simulink model "IM_close-loop"  (R2019a)
settings: Solver=FixedStepAuto  StartTime=0.0  StopTime=1  FixedStep=0.00001  RelTol=1e-3
values from neighbouring files (symbols this model uses):
  A1 = [a1 0 a2 0; 0 a1 0 a2; a4 0 a5 0 ; 0 a4 0 a5]    [parametre_IM.m]
  A2 = [0 0 0 a3; 0 0 -a3 0 ; 0 0 0 -1 ; 0 0 1 0]    [parametre_IM.m]
  B = [1/(Ls*sigma) 0; 0 1/(Ls*sigma); 0 0; 0 0]    [parametre_IM.m]
  ClarkConcordia = sqrt(3/2)*[1 -1/2 -1/2; 0 sqrt(3)/2 -sqrt(3)/2; 1/sqrt(2) 1/sqrt(2) 1/sqrt(2)]    [parametre_IM.m]
  ctevf = 240/(2*pi*50)    (= 0.763943726841)    [parametre_IM.m]
  f = 0    [parametre_IM.m]
  fpr = 1000    [parametre_IM.m]
  J = 0.07    [parametre_IM.m]
  Lr = 0.1568    [parametre_IM.m]
  M = 0.15    [parametre_IM.m]
  p = 2    [parametre_IM.m]
  T = [2/3 -1/3 -1/3; -1/3 2/3 -1/3; -1/3 -1/3 2/3]    [parametre_IM.m]
libraries: simulink x2
settings Model: Creator=TOSHIBA  LastModifiedBy=TOSHIBA

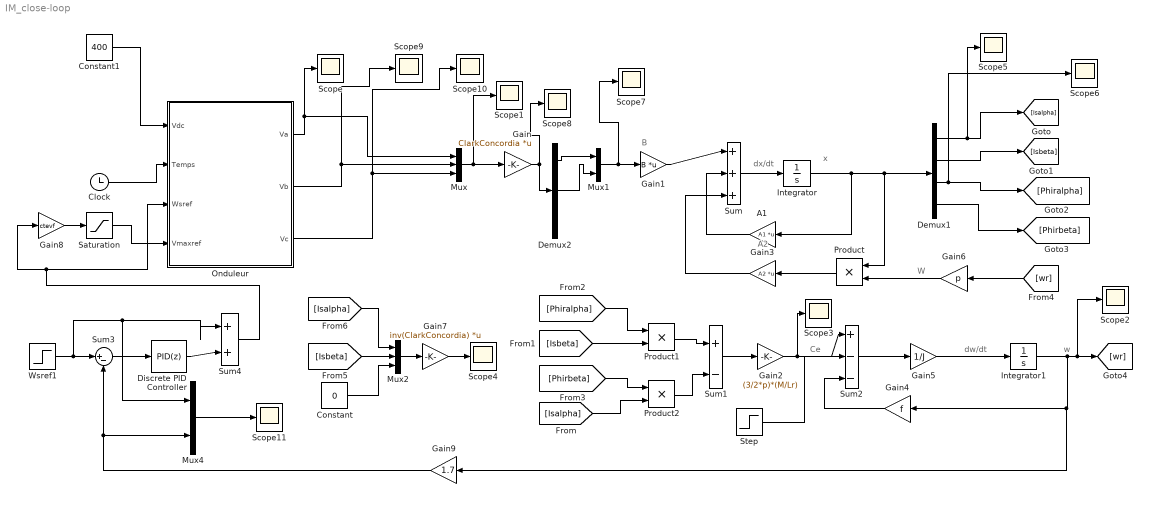
== system IM_close-loop ==
  note: W
  note: w
  note: dw/dt
  note: Ce
  note: A2
  note: B
  note: x
  note: dx/dt
  A1 : Gain  Gain=A1  Multiplication=Matrix(K*u)
  Clock : Clock
  Constant : Constant  Value=0
  Constant1 : Constant  Value=400
  Demux1 : Demux
  Demux2 : Demux  Outputs=3
  Discrete PID Controller : simulink/Continuous/PID Controller  Controller=PID  Form=Parallel  TimeDomain=Discrete-time  SampleTime=-1  IntegratorMethod=Forward Euler  FilterMethod=Forward Euler  ControllerParametersSource=internal  P=0.01  I=0.003  D=0  UseFilter=on  N=100  TunerSelectOption=Transfer Function Based (PID Tuner App)  InitialConditionSource=internal  InitialConditionForIntegrator=0  InitialConditionForFilter=0  DifferentiatorICPrevScaledInput=0  ExternalReset=none  TrackingMode=off  Kt=1  LimitOutput=off  UpperSaturationLimit=inf  LowerSaturationLimit=-inf  LinearizeAsGain=off  AntiWindupMode=none  Kb=1  POutMin=[]  POutMax=[]  IOutMin=[]  IOutMax=[]  DOutMin=[]  DOutMax=[]  NOutMin=[]  NOutMax=[]  SumOutMin=[]  SumOutMax=[]  SaturationOutMin=[]  SaturationOutMax=[]  PParamMin=[]  PParamMax=[]  IParamMin=[]  IParamMax=[]  DParamMin=[]  DParamMax=[]  NParamMin=[]  NParamMax=[]  KbParamMin=[]  KbParamMax=[]  KtParamMin=[]  KtParamMax=[]  KbOutMin=[]  KbOutMax=[]  KtOutMin=[]  KtOutMax=[]  IntegratorOutMin=[]  IntegratorOutMax=[]  FilterOutMin=[]  FilterOutMax=[]  SumI1OutMin=[]  SumI1OutMax=[]  SumI2OutMin=[]  SumI2OutMax=[]  SumI3OutMin=[]  SumI3OutMax=[]  SumI4OutMin=[]  SumI4OutMax=[]  SumDOutMin=[]  SumDOutMax=[]  DifferentiatorOutMin=[]  DifferentiatorOutMax=[]  FilterDiffOutCoefMin=[]  FilterDiffOutCoefMax=[]  ReciprocalOutMin=[]  ReciprocalOutMax=[]  SumDenOutMin=[]  SumDenOutMax=[]  SumNumOutMin=[]  SumNumOutMax=[]  DivideOutMin=[]  DivideOutMax=[]  IntegratorContinuousStateAttributes=''  IntegratorStateMustResolveToSignalObject=off  IntegratorRTWStateStorageClass=Auto  FilterContinuousStateAttributes=''  FilterStateMustResolveToSignalObject=off  FilterRTWStateStorageClass=Auto  ParallelPVariant=InternalParameters  IdealPVariant=Disabled  IVariant=InternalParameters  DVariant=InternalParameters  IntegratorVariant=Discrete  SatVariant=Disabled  AWVariant=Passthrough  PCopyVariant=Disabled  TRVariant=Disabled  FdbkBlocksVariant=Forward  IdealPFdbkVariant=Disabled  SatFdbkVariant=Disabled  DerivativeFilterVariant=ForwardEulerFilter  NVariant=InternalParameters  NCopyVariant=Disabled  FilterICVariant=InternalICsFilter  IntegratorICVariant=InternalICs  ExternalResetVariant=Disabled  TRSumVariant=Passthrough  SumFdbkVariant=Disabled  SumVariant=Sum_PID
  Gain : Gain  Gain=ClarkConcordia  Multiplication=Matrix(K*u)
  Gain1 : Gain  Gain=B  Multiplication=Matrix(K*u)
  Gain2 : Gain  Gain=(3/2*p)*(M/Lr)
  Gain3 : Gain  Gain=A2  Multiplication=Matrix(K*u)
  Gain4 : Gain  Gain=f
  Gain5 : Gain  Gain=1/J
  Gain6 : Gain  Gain=p
  Gain7 : Gain  Gain=inv(ClarkConcordia)  Multiplication=Matrix(K*u)
  Gain8 : Gain  Gain=ctevf
  Gain9 : Gain  Gain=1.7
  Integrator : Integrator
  Integrator1 : Integrator
  Mux : Mux  Inputs=3
  Mux1 : Mux  Inputs=2
  Mux2 : Mux  Inputs=3
  Mux4 : Mux  Inputs=2
  Onduleur : Subsystem
  Product : Product
  Product1 : Product
  Product2 : Product
  Saturation : Saturate  UpperLimit=500
  Scope{,1..11} (12 alike) : Scope
  Step : Step  Time=0  After=0  SampleTime=0
  Sum : Sum  Inputs=|+++
  Sum1 : Sum  Inputs=|+-
  Sum2 : Sum  Inputs=|+--
  Sum3 : Sum  Inputs=|+-
  Sum4 : Sum  Inputs=|++
  Wsref1 : Step  Time=0.5  Before=2*pi*50  After=2*pi*100  SampleTime=0
  wires:
  Onduleur/1("Va ") -> Mux/1, Scope/1
  Onduleur/2(Vb) -> Mux/2, Scope9/1
  Onduleur/3(Vc) -> Mux/3, Scope10/1
  Mux/1 -> Scope1/1, Gain/1
  Mux1/1 -> Scope7/1, Gain1/1
  Sum/1 -> Integrator/1
  Gain1/1 -> Sum/1
  A1/1 -> Sum/2
  Gain3/1 -> Sum/3
  Integrator/1 -> A1/1, Product/1, Demux1/1
  Product/1 -> Gain3/1
  Demux1/1 -> Scope5/1, [Isalpha]
  Demux1/2 -> [Isbeta]
  Demux1/3 -> Scope6/1, [Phiralpha]
  Demux1/4 -> [Phirbeta]
  [Phiralpha] -> Product1/1
  [Isbeta] -> Product1/2
  [Phirbeta] -> Product2/1
  [Isalpha] -> Product2/2
  Product1/1 -> Sum1/1
  Product2/1 -> Sum1/2
  Sum1/1 -> Gain2/1
  Gain2/1 -> Scope3/1, Sum2/1
  Step/1 -> Sum2/2
  Gain4/1 -> Sum2/3
  Sum2/1 -> Gain5/1
  Gain5/1 -> Integrator1/1
  Integrator1/1 -> Scope2/1, [wr], Gain9/1, Gain4/1
  [wr] -> Gain6/1
  Gain6/1 -> Product/2
  Gain7/1 -> Scope4/1
  Mux2/1 -> Gain7/1
  [Isalpha] -> Mux2/1
  [Isbeta] -> Mux2/2
  Constant/1 -> Mux2/3
  Demux2/1 -> Mux1/1
  Demux2/2 -> Mux1/2
  Gain/1 -> Scope8/1, Demux2/1
  Clock/1 -> Onduleur/2(Temps)
  Discrete PID Controller/1 -> Sum4/2
  Constant1/1 -> Onduleur/1(Vdc)
  Gain8/1 -> Saturation/1
  Saturation/1 -> Onduleur/4("Vmaxref ")
  Wsref1/1 -> Mux4/1, Sum4/1, Sum3/1
  Sum3/1 -> Discrete PID Controller/1
  Sum4/1 -> Gain8/1, Onduleur/3(Wsref)
  Mux4/1 -> Scope11/1
  Gain9/1 -> Sum3/2, Mux4/2

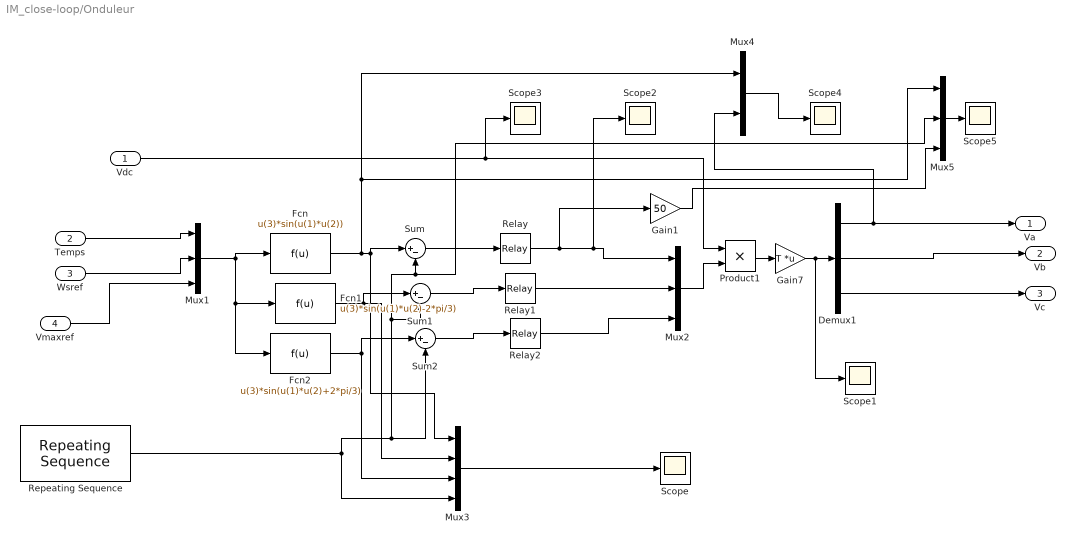
== system IM_close-loop/Onduleur ==
  Vdc : Inport
  Temps : Inport  Port=2
  Wsref : Inport  Port=3
  "Vmaxref " : Inport  Port=4
  Demux1 : Demux  Outputs=3
  Fcn : Fcn  Expr=u(3)*sin(u(1)*u(2))
  Fcn1 : Fcn  Expr=u(3)*sin(u(1)*u(2)-2*pi/3)
  Fcn2 : Fcn  Expr=u(3)*sin(u(1)*u(2)+2*pi/3)
  Gain1 : Gain  Gain=50
  Gain7 : Gain  Gain=T  Multiplication=Matrix(K*u)
  Mux1 : Mux  Inputs=3
  Mux2 : Mux  Inputs=3
  Mux3 : Mux
  Mux4 : Mux  Inputs=2
  Mux5 : Mux  Inputs=3
  Product1 : Product
  Relay : Relay  OffOutputValue=-1
  Relay1 : Relay  OffOutputValue=-1
  Relay2 : Relay  OffOutputValue=-1
  Repeating Sequence : simulink/Sources/Repeating Sequence  rep_seq_t=[0 1/(2*fpr) 1/fpr]  rep_seq_y=[-400 400 -400]
  Scope{,1..5} (6 alike) : Scope
  Sum : Sum  Inputs=|+-
  Sum1 : Sum  Inputs=|+-
  Sum2 : Sum  Inputs=|+-
  "Va " : Outport
  Vb : Outport  Port=2
  Vc : Outport  Port=3
  wires:
  Repeating Sequence/1 -> Mux5/2, Sum/2, Sum1/2, Sum2/2, Mux3/4
  Mux2/1 -> Product1/2
  Mux1/1 -> Fcn2/1, Fcn1/1, Fcn/1
  Demux1/1 -> Mux4/2, "Va "/1
  Relay/1 -> Gain1/1, Scope2/1, Mux2/1
  Gain7/1 -> Scope1/1, Demux1/1
  Relay1/1 -> Mux2/2
  Sum/1 -> Relay/1
  Demux1/3 -> Vc/1
  Sum1/1 -> Relay1/1
  Fcn2/1 -> Sum2/1, Mux3/3
  Fcn1/1 -> Mux3/2, Sum1/1
  Fcn/1 -> Mux5/1, Mux4/1, Mux3/1, Sum/1
  Product1/1 -> Gain7/1
  Relay2/1 -> Mux2/3
  Vdc/1 -> Scope3/1, Product1/1
  Sum2/1 -> Relay2/1
  Wsref/1 -> Mux1/2
  Temps/1 -> Mux1/1
  Demux1/2 -> Vb/1
  Mux3/1 -> Scope/1
  "Vmaxref "/1 -> Mux1/3
  Mux4/1 -> Scope4/1
  Gain1/1 -> Mux5/3
  Mux5/1 -> Scope5/1
